simulink model "BarrierLog"  (R2021a)
settings: Solver=ode1  StartTime=0.0  StopTime=80  FixedStep=0.001  RelTol=1e-3  EnableMultiTasking=on
values from neighbouring files (symbols this model uses):
  alpha1 = 2    [gains.m]
  alpha2 = 2    [gains.m]
  initialValues = [ 0 0 0 0 0]    [gains.m]
  Ke1 = 2    [gains.m]
  Ke2 = 2    [gains.m]
  Kr1 = 50    [gains.m]
  Kr2 = 50    [gains.m]
settings Model: Creator=ezergeroglu  LastModifiedBy=Mesih
settings SolverCC: AlgebraicLoopSolver=TrustRegion
settings DataIOCC: LimitDataPoints=on  SaveFormat=Array  SignalLoggingSaveFormat=ModelDataLogs  ReturnWorkspaceOutputs=off  SignalLoggingName=sigsOut
settings OptimizationCC: BooleanDataType=off
settings DebuggingCC: SaveWithParameterizedLinksMsg=none  UnderspecifiedInitializationDetection=Classic  MergeDetectMultiDrivingBlocksExec=none  SignalResolutionControl=TryResolveAllWithWarning  MultiTaskDSMMsg=warning  MultiTaskCondExecSysMsg=none  SFMachineParentedDataDiag=warning  ArithmeticOperatorsInVariantConditions=warning
settings HardwareCC: ProdBitPerPointer=32  ProdBitPerSizeT=32  ProdBitPerPtrDiffT=32  ProdLargestAtomicFloat=None  ProdIntDivRoundTo=Undefined  ProdEndianess=Unspecified  ProdWordSize=32  ProdHWDeviceType=32-bit Generic  TargetUnknown=on
settings ModelReferenceCC: PropagateSignalLabelsOutOfModel=off
settings SFSimCC: SimUseLocalCustomCode=off  CustomCodeUndefinedFunction=UseInterfaceOnly
settings RTWCC: RTWUseLocalCustomCode=off
settings CodeAppCC: StateflowObjectComments=on
settings GRTTargetCC: TargetLangStandard=C89/C90 (ANSI)  CombineOutputUpdateFcns=off  GRTInterface=on
settings ConfigComp: CovMetricSettings=dw  CovSaveCumulativeToWorkspaceVar=on  CovSaveSingleToWorkspaceVar=on  CovExternalEMLEnable=off

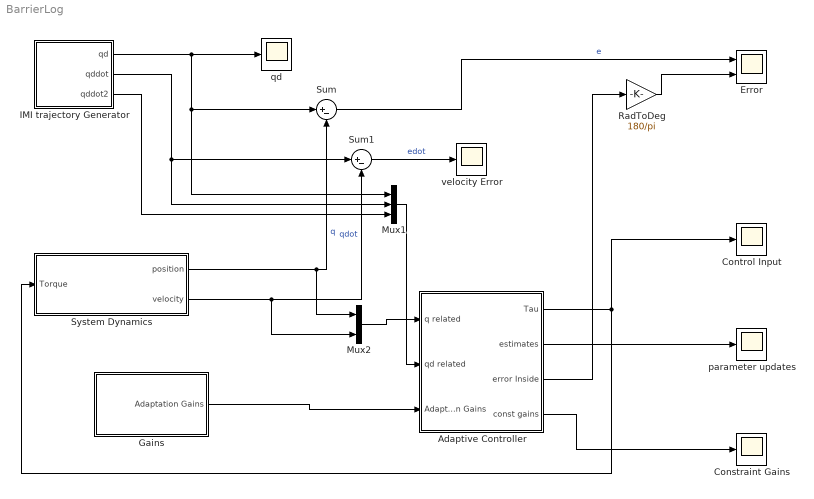
== system BarrierLog ==
  Adaptive Controller : Subsystem
  Constraint Gains : Scope
  Control Input : Scope
  Error : Scope  NumInputPorts=2
  Gains : Subsystem
  IMI trajectory Generator : Subsystem  mask{ampl=[0.7  1.2], freq=[1.0 1.0]}
      mask prompts: ampl "Amplitute"; freq "Frequency"
  Mux1 : Mux  Inputs=3
  Mux2 : Mux  Inputs=2
  RadToDeg : Gain  Gain=180/pi  SaturateOnIntegerOverflow=on  OutDataTypeStr=Inherit: Same as input  ParamDataTypeStr=Inherit: Same as input
  Sum : Sum  Inputs=|+-  InputSameDT=on  SaturateOnIntegerOverflow=on  OutDataTypeStr=Inherit: Same as first input
  Sum1 : Sum  Inputs=|+-  InputSameDT=on  SaturateOnIntegerOverflow=on  OutDataTypeStr=Inherit: Same as first input
  System Dynamics : Subsystem
  parameter updates : Scope
  qd : Scope
  velocity Error : Scope
  wires:
  Sum/1 -> Error/1  "e"
  System Dynamics/1(position) -> Sum/2, Mux2/1  "q"
  System Dynamics/2(velocity) -> Sum1/2, Mux2/2  "qdot"
  Sum1/1 -> velocity Error/1  "edot"
  Adaptive Controller/1(Tau) -> System Dynamics/1(Torque), Control Input/1
  Mux1/1 -> Adaptive Controller/2(qd related)
  Mux2/1 -> Adaptive Controller/1(q related)
  Adaptive Controller/2(estimates) -> parameter updates/1
  Adaptive Controller/3(error Inside) -> RadToDeg/1
  Gains/1(Adaptation Gains) -> Adaptive Controller/3(Adaptation Gains)
  IMI trajectory Generator/1(qd) -> Sum/1, Mux1/1, qd/1
  IMI trajectory Generator/2(qddot) -> Sum1/1, Mux1/2
  IMI trajectory Generator/3(qddot2) -> Mux1/3
  RadToDeg/1 -> Error/2
  Adaptive Controller/4(const gains) -> Constraint Gains/1

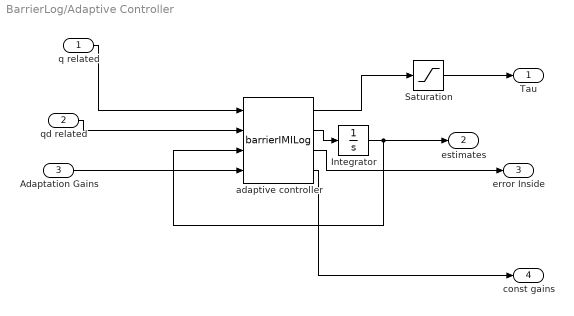
== system BarrierLog/Adaptive Controller ==
  q related : Inport
  qd related : Inport  Port=2
  Adaptation Gains : Inport  Port=3
  Integrator : Integrator  InitialCondition=initialValues
  Saturation : Saturate  UpperLimit=10  LowerLimit=-10
  adaptive controller : S-Function  FunctionName=barrierIMILog  Parameters=[Kr1, Kr2], [alpha1, alpha2], [Ke1, Ke2]  SFunctionDeploymentMode=off  EnableBusSupport=off
  Tau : Outport  VectorParamsAs1DForOutWhenUnconnected=off
  estimates : Outport  Port=2  VectorParamsAs1DForOutWhenUnconnected=off
  error Inside : Outport  Port=3  VectorParamsAs1DForOutWhenUnconnected=off
  const gains : Outport  Port=4
  wires:
  q related/1 -> adaptive controller/1
  adaptive controller/1 -> Saturation/1
  qd related/1 -> adaptive controller/2
  adaptive controller/3 -> error Inside/1
  adaptive controller/2 -> Integrator/1
  Integrator/1 -> estimates/1, adaptive controller/3
  Adaptation Gains/1 -> adaptive controller/4
  Saturation/1 -> Tau/1
  adaptive controller/4 -> const gains/1

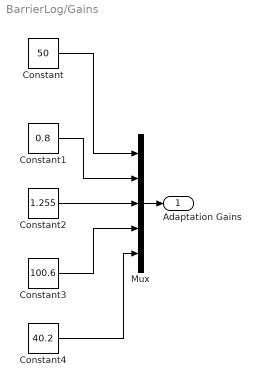
== system BarrierLog/Gains ==
  Constant : Constant  Value=50
  Constant1 : Constant  Value=0.8
  Constant2 : Constant  Value=1.255
  Constant3 : Constant  Value=100.6
  Constant4 : Constant  Value=40.2
  Mux : Mux  Inputs=5
  Adaptation Gains : Outport  VectorParamsAs1DForOutWhenUnconnected=off
  wires:
  Mux/1 -> Adaptation Gains/1
  Constant/1 -> Mux/1
  Constant1/1 -> Mux/2
  Constant2/1 -> Mux/3
  Constant3/1 -> Mux/4
  Constant4/1 -> Mux/5

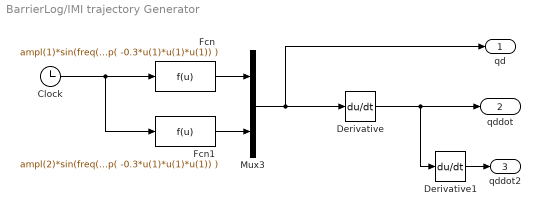
== system BarrierLog/IMI trajectory Generator ==
  Clock : Clock
  Derivative : Derivative
  Derivative1 : Derivative
  Fcn : Fcn  Expr=ampl(1)*sin(freq(1)*u(1))*( 1-exp( -0.3*u(1)*u(1)*u(1)) )
  Fcn1 : Fcn  Expr=ampl(2)*sin(freq(2)*u(1))*( 1-exp( -0.3*u(1)*u(1)*u(1)) )
  Mux3 : Mux  Inputs=2
  qd : Outport  VectorParamsAs1DForOutWhenUnconnected=off
  qddot : Outport  Port=2  VectorParamsAs1DForOutWhenUnconnected=off
  qddot2 : Outport  Port=3  VectorParamsAs1DForOutWhenUnconnected=off
  wires:
  Clock/1 -> Fcn/1, Fcn1/1
  Fcn/1 -> Mux3/1
  Fcn1/1 -> Mux3/2
  Mux3/1 -> Derivative/1, qd/1
  Derivative/1 -> Derivative1/1, qddot/1
  Derivative1/1 -> qddot2/1

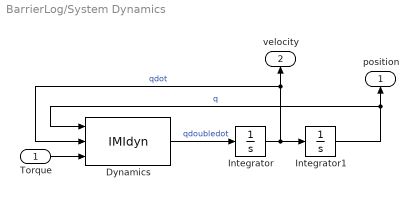
== system BarrierLog/System Dynamics ==
  Torque : Inport
  Dynamics : S-Function  FunctionName=IMIdyn  SFunctionDeploymentMode=off  EnableBusSupport=off
  Integrator : Integrator
  Integrator1 : Integrator  InitialCondition=2.9*pi/180
  position : Outport  VectorParamsAs1DForOutWhenUnconnected=off
  velocity : Outport  Port=2  VectorParamsAs1DForOutWhenUnconnected=off
  wires:
  Dynamics/1 -> Integrator/1  "qdoubledot"
  Integrator/1 -> Integrator1/1, velocity/1, Dynamics/2  "qdot"
  Integrator1/1 -> position/1, Dynamics/1  "q"
  Torque/1 -> Dynamics/3
